simulink model "Copy_of_step_response"  (R2022a)
settings: Solver=VariableStepAuto  StartTime=0.0  StopTime=1000.0  RelTol=1e-3
settings Model: Creator=SPY  LastModifiedBy=SPY

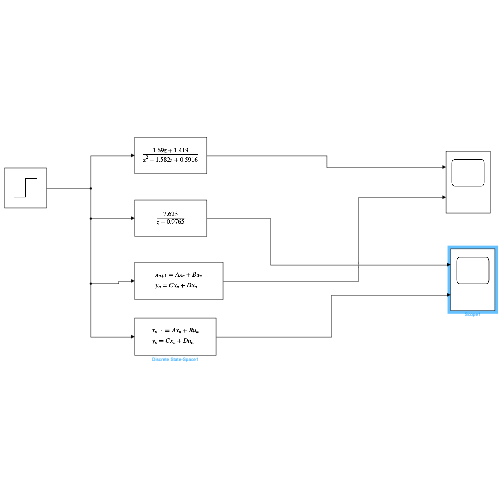
[thumbnail: Simulink's stored preview of the top-level diagram]
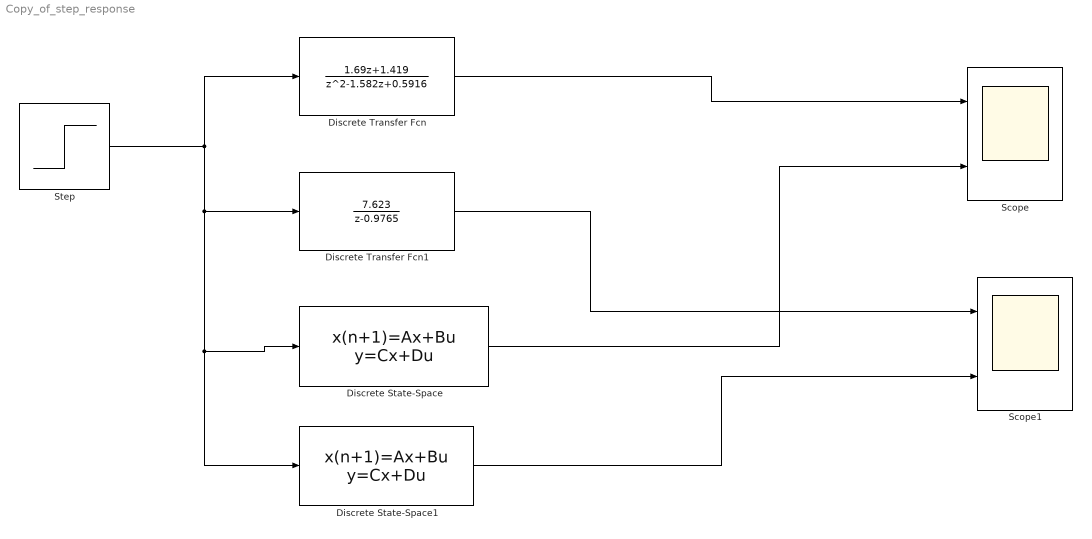
== system Copy_of_step_response ==
  Discrete Transfer Fcn : DiscreteTransferFcn  Numerator=[1.69 1.419]  Denominator=[1 -1.582 0.5916]
  Discrete Transfer Fcn1 : DiscreteTransferFcn  Numerator=[7.623]  Denominator=[1 -0.9765]  SampleTime=1
  Discrete State-Space : DiscreteStateSpace  A=[1.582 -0.5916; 1 0]  B=[1; 0]  C=[1.69 1.419]  D=0  SampleTime=-1
  Discrete State-Space1 : DiscreteStateSpace  A=0.9765  C=7.6230  D=0
  Scope : Scope  NumInputPorts=2
  Scope1 : Scope  NumInputPorts=2
  Step : Step  SampleTime=5
  wires:
  Step/1 -> Discrete Transfer Fcn/1, Discrete State-Space1/1, Discrete State-Space/1, Discrete Transfer Fcn1/1
  Discrete Transfer Fcn/1 -> Scope/1
  Discrete State-Space/1 -> Scope/2
  Discrete Transfer Fcn1/1 -> Scope1/1
  Discrete State-Space1/1 -> Scope1/2
